simulink library "rocket_dynamic_data_library"  (R2014a)
settings: Solver=ode45  StartTime=0.0  StopTime=10.0  RelTol=1e-3
settings Model: Creator=scorpii  LastModifiedBy=scorpii

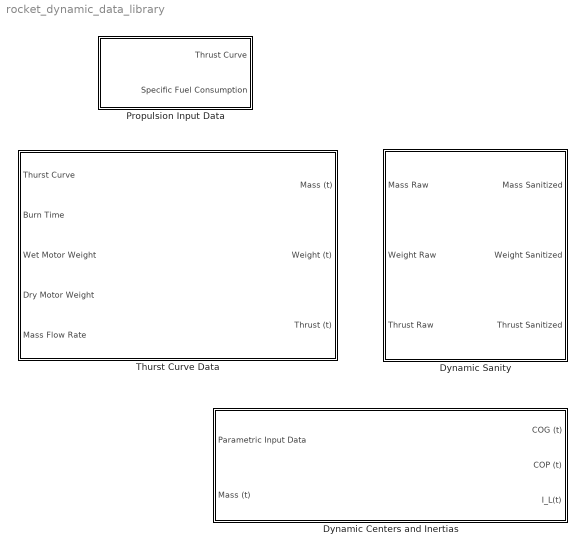
== system rocket_dynamic_data_library ==
  Dynamic Centers and Inertias : Subsystem
  Dynamic Sanity : Subsystem
  Propulsion Input Data : Subsystem
  Thurst Curve Data : Subsystem

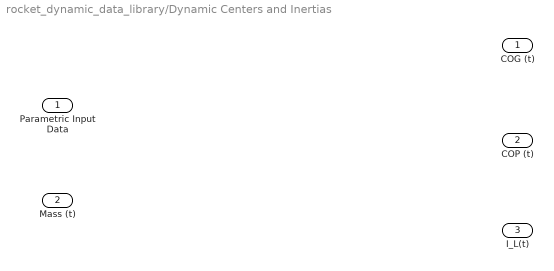
== system rocket_dynamic_data_library/Dynamic Centers and Inertias ==
  Parametric Input Data : Inport
  Mass (t) : Inport  Port=2
  COG (t) : Outport
  COP (t) : Outport  Port=2
  I_L(t) : Outport  Port=3

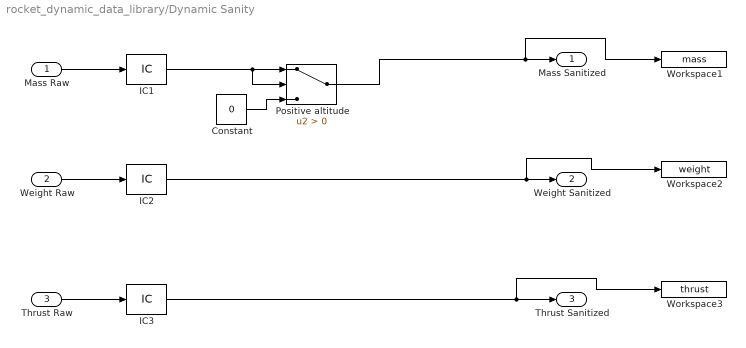
== system rocket_dynamic_data_library/Dynamic Sanity ==
  Mass Raw : Inport
  Weight Raw : Inport  Port=2
  Thrust Raw : Inport  Port=3
  Constant : Constant  Value=0
  IC1 : InitialCondition  Value=0
  IC2 : InitialCondition  Value=0
  IC3 : InitialCondition  Value=0
  Positive altitude : Switch  Criteria=u2 > Threshold
  Workspace1 : ToWorkspace  VariableName=mass  SampleTime=-1
  Workspace2 : ToWorkspace  VariableName=weight  SampleTime=-1
  Workspace3 : ToWorkspace  VariableName=thrust  SampleTime=-1
  Mass Sanitized : Outport
  Weight Sanitized : Outport  Port=2
  Thrust Sanitized : Outport  Port=3
  wires:
  Constant/1 -> Positive altitude/3
  Weight Raw/1 -> IC2/1
  Positive altitude/1 -> Workspace1/1, Mass Sanitized/1
  Thrust Raw/1 -> IC3/1
  Mass Raw/1 -> IC1/1
  IC1/1 -> Positive altitude/2, Positive altitude/1
  IC2/1 -> Workspace2/1, Weight Sanitized/1
  IC3/1 -> Workspace3/1, Thrust Sanitized/1

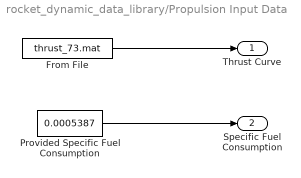
== system rocket_dynamic_data_library/Propulsion Input Data ==
  From File : FromFile  FileName=thrust_73.mat  OutDataTypeStr=double  ExtrapolationAfterLastDataPoint=Ground value
  Provided Specific Fuel Consumption : Constant  Value=0.0005387
  Thrust Curve : Outport
  Specific Fuel Consumption : Outport  Port=2
  wires:
  Provided Specific Fuel Consumption/1 -> Specific Fuel Consumption/1
  From File/1 -> Thrust Curve/1

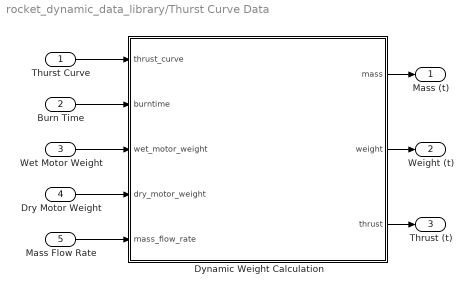
== system rocket_dynamic_data_library/Thurst Curve Data ==
  Thurst Curve : Inport
  Burn Time : Inport  Port=2
  Wet Motor Weight : Inport  Port=3
  Dry Motor Weight : Inport  Port=4
  Mass Flow Rate : Inport  Port=5
  Dynamic Weight Calculation : Subsystem
  Mass (t) : Outport
  Weight (t) : Outport  Port=2
  "Thrust (t) " : Outport  Port=3
  wires:
  Thurst Curve/1 -> Dynamic Weight Calculation/1(thrust_curve)
  Wet Motor Weight/1 -> Dynamic Weight Calculation/3(wet_motor_weight)
  Mass Flow Rate/1 -> Dynamic Weight Calculation/5(mass_flow_rate)
  Dynamic Weight Calculation/1(mass) -> Mass (t)/1
  Dynamic Weight Calculation/2(weight) -> Weight (t)/1
  Dynamic Weight Calculation/3(thrust) -> "Thrust (t) "/1
  Burn Time/1 -> Dynamic Weight Calculation/2(burntime)
  Dry Motor Weight/1 -> Dynamic Weight Calculation/4(dry_motor_weight)

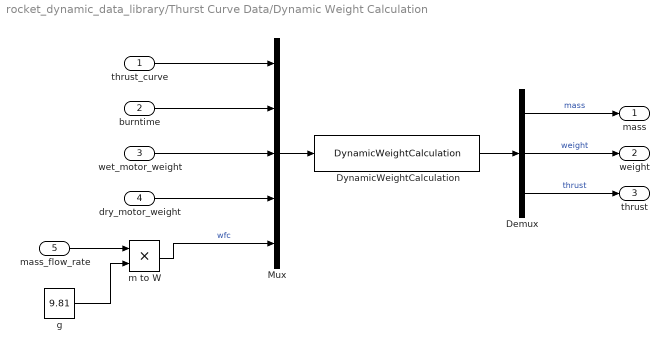
== system rocket_dynamic_data_library/Thurst Curve Data/Dynamic Weight Calculation ==
  thrust_curve : Inport
  burntime : Inport  Port=2
  wet_motor_weight : Inport  Port=3
  dry_motor_weight : Inport  Port=4
  mass_flow_rate : Inport  Port=5
  Demux : Demux  Outputs=[1 1 1]
  DynamicWeightCalculation : MATLABFcn  MATLABFcn=DynamicWeightCalculation
      mask Display: disp('DynamicWeightCalculation')
  Mux : Mux  Inputs=5
  g : Constant  Value=9.81
  m to W : Product
  mass : Outport
  weight : Outport  Port=2
  thrust : Outport  Port=3
  wires:
  burntime/1 -> Mux/2
  Demux/1 -> mass/1  "mass"
  Demux/2 -> weight/1  "weight"
  Mux/1 -> DynamicWeightCalculation/1
  DynamicWeightCalculation/1 -> Demux/1
  Demux/3 -> thrust/1  "thrust"
  mass_flow_rate/1 -> m to W/1
  g/1 -> m to W/2
  m to W/1 -> Mux/5  "wfc"
  wet_motor_weight/1 -> Mux/3
  thrust_curve/1 -> Mux/1
  dry_motor_weight/1 -> Mux/4
